simulink model "celsiusConverter_Rafael_Enriquezslx"  (R2022b)
settings: Solver=VariableStepAuto  StartTime=0.0  StopTime=10.0  RelTol=1e-3
settings Model: Creator=fitir  LastModifiedBy=fitir

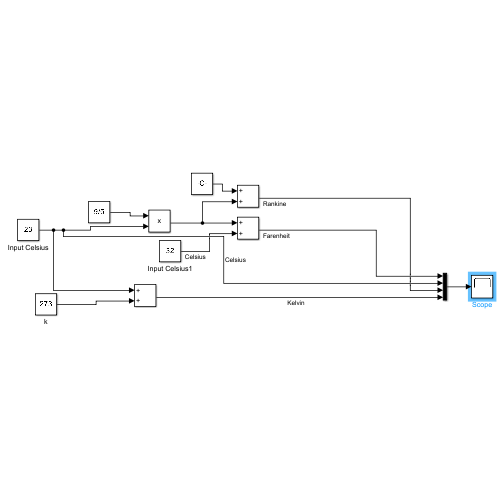
[thumbnail: Simulink's stored preview of the top-level diagram]
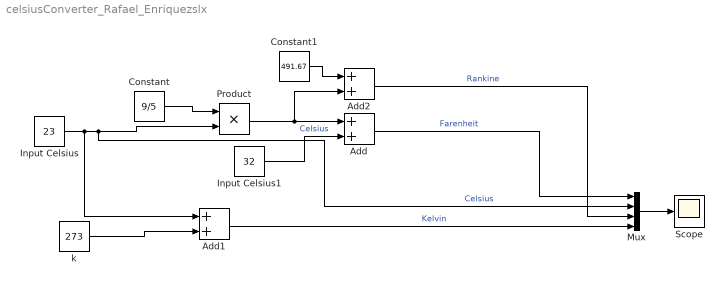
== system celsiusConverter_Rafael_Enriquezslx ==
  Add : Sum
  Add1 : Sum
  Add2 : Sum
  Constant : Constant  Value=9/5
  Constant1 : Constant  Value=491.67
  Input Celsius : Constant  Value=23  SampleTime=1
  Input Celsius1 : Constant  Value=32  SampleTime=1
  Mux : Mux
  Product : Product
  Scope : Scope
  k : Constant  Value=273  SampleTime=1
  wires:
  Mux/1 -> Scope/1
  Input Celsius/1 -> Add1/1, Product/2, Mux/2  "Celsius"
  Constant/1 -> Product/1
  Product/1 -> Add2/2, Add/1
  Input Celsius1/1 -> Add/2  "Celsius"
  Add/1 -> Mux/1  "Farenheit"
  k/1 -> Add1/2
  Add1/1 -> Mux/4  "Kelvin"
  Add2/1 -> Mux/3  "Rankine"
  Constant1/1 -> Add2/1
